simulink model "SingleTrack"  (Simulink 8.7)
settings: Solver=ode45  SolverMode=SingleTasking  StartTime=0.0  StopTime=inf  FixedStep=0.001  RelTol=1e-3
PreLoadFcn:
  | SingleTrack_params
undefined symbols (not defined in the file): Car_Bdy1_mass, Car_Steering_i, Car_Whl_Radius, Car_WhlBaseF, Car_WhlBaseR, mEngineMax, PT_DL_iDiff, PT_GearBox_iForwardGears
libraries: CarMaker4SL x7
(part 3 of 4)

== system SingleTrack/CarMaker/Vehicle/IPG Vehicle/CarAndTrailer/Forces/Tires ==
  note: The TireXX_Out signals will only be used if FileIdent is "CarMaker-Tire-CM4SL" in the tire parameter file!
      | An example parameter file can be found in Data/Tire/DT_CM4SL_UserTire.
  Sync_In : Inport
  TireFL_In : Inport  Port=2
  TireFR_In : Inport  Port=3
  TireRL_In : Inport  Port=4
  TireRR_In : Inport  Port=5
  Bus Creator{1..4} (4 alike) : BusCreator  Inputs=11
  Demux{1..3,8} (4 alike) : Demux  Outputs=7
  TireFL : Subsystem
  TireFR : Subsystem
  TireRL : Subsystem
  TireRR : Subsystem
  TireFL_Out : Outport
  TireFR_Out : Outport  Port=2
  TireRL_Out : Outport  Port=3
  TireRR_Out : Outport  Port=4
  wires:
  Sync_In/1 -> TireRR/1(Sync_In), TireRL/1(Sync_In), TireFR/1(Sync_In), TireFL/1(Sync_In)
  Bus Creator4/1 -> TireRR_Out/1
  Bus Creator2/1 -> TireRL_Out/1
  Bus Creator1/1 -> TireFR_Out/1
  Demux3/5 -> TireRR/6(Rim_turnv)  "Tire_In Rim_turnv"
  Demux3/4 -> TireRR/5(Rim_rotv)  "Tire_In Rim_rotv"
  Demux3/1 -> TireRR/2(Load)  "Tire_In Load"
  Demux3/7 -> TireRR/8(muRoad)  "Tire_In mu"
  Demux3/6 -> TireRR/7(InclinAngle)  "Tire_In Camber"
  Demux3/2 -> TireRR/3(vxtrans)  "Tire_In vxtrans"
  Demux3/3 -> TireRR/4(vytrans)  "Tire_In vytrans"
  TireRR/11(AlignTrq) -> Bus Creator4/11  "Tire_Out AlignTrq"
  TireRR/10(RollResist) -> Bus Creator4/10  "Tire_Out RollResist"
  TireRR/9(OverturnTrq) -> Bus Creator4/9  "Tire_Out OverturnTrq"
  TireRR/8(LoadFrc) -> Bus Creator4/8  "Tire_Out LoadFrc"
  TireRR/7(SideFrc) -> Bus Creator4/7  "Tire_Out SideFrc"
  TireRR/6(LongFrc) -> Bus Creator4/6  "Tire_Out LongFrc"
  TireRR/5(vBelt) -> Bus Creator4/5  "Tire_Out vBelt"
  TireRR/4(rBelt_eff) -> Bus Creator4/4  "Tire_Out rBelt_eff"
  TireRR/3(TurnSlp) -> Bus Creator4/3  "Tire_Out TurnSlp"
  TireRR/1(Slp) -> Bus Creator4/1  "Tire_Out Slp"
  TireRR/2(Alpha) -> Bus Creator4/2  "Tire_Out Alpha"
  Demux2/5 -> TireRL/6(Rim_turnv)  "Tire_In Rim_turnv"
  Demux2/4 -> TireRL/5(Rim_rotv)  "Tire_In Rim_rotv"
  Demux2/1 -> TireRL/2(Load)  "Tire_In Load"
  Demux2/7 -> TireRL/8(muRoad)  "Tire_In mu"
  Demux2/6 -> TireRL/7(InclinAngle)  "Tire_In Camber"
  Demux2/2 -> TireRL/3(vxtrans)  "Tire_In vxtrans"
  Demux2/3 -> TireRL/4(vytrans)  "Tire_In vytrans"
  TireRL/11(AlignTrq) -> Bus Creator2/11  "Tire_Out AlignTrq"
  TireRL/10(RollResist) -> Bus Creator2/10  "Tire_Out RollResist"
  TireRL/9(OverturnTrq) -> Bus Creator2/9  "Tire_Out OverturnTrq"
  TireRL/8(LoadFrc) -> Bus Creator2/8  "Tire_Out LoadFrc"
  TireRL/7(SideFrc) -> Bus Creator2/7  "Tire_Out SideFrc"
  TireRL/6(LongFrc) -> Bus Creator2/6  "Tire_Out LongFrc"
  TireRL/5(vBelt) -> Bus Creator2/5  "Tire_Out vBelt"
  TireRL/4(rBelt_eff) -> Bus Creator2/4  "Tire_Out rBelt_eff"
  TireRL/3(TurnSlp) -> Bus Creator2/3  "Tire_Out TurnSlp"
  TireRL/1(Slp) -> Bus Creator2/1  "Tire_Out Slp"
  TireRL/2(Alpha) -> Bus Creator2/2  "Tire_Out Alpha"
  Demux1/5 -> TireFR/6(Rim_turnv)  "Tire_In Rim_turnv"
  Demux1/4 -> TireFR/5(Rim_rotv)  "Tire_In Rim_rotv"
  Demux1/1 -> TireFR/2(Load)  "Tire_In Load"
  Demux1/7 -> TireFR/8(muRoad)  "Tire_In mu"
  Demux1/6 -> TireFR/7(InclinAngle)  "Tire_In Camber"
  Demux1/2 -> TireFR/3(vxtrans)  "Tire_In vxtrans"
  Demux1/3 -> TireFR/4(vytrans)  "Tire_In vytrans"
  TireFR/11(AlignTrq) -> Bus Creator1/11  "Tire_Out AlignTrq"
  TireFR/10(RollResist) -> Bus Creator1/10  "Tire_Out RollResist"
  TireFR/9(OverturnTrq) -> Bus Creator1/9  "Tire_Out OverturnTrq"
  TireFR/8(LoadFrc) -> Bus Creator1/8  "Tire_Out LoadFrc"
  TireFR/7(SideFrc) -> Bus Creator1/7  "Tire_Out SideFrc"
  TireFR/6(LongFrc) -> Bus Creator1/6  "Tire_Out LongFrc"
  TireFR/5(vBelt) -> Bus Creator1/5  "Tire_Out vBelt"
  TireFR/4(rBelt_eff) -> Bus Creator1/4  "Tire_Out rBelt_eff"
  TireFR/3(TurnSlp) -> Bus Creator1/3  "Tire_Out TurnSlp"
  TireFR/1(Slp) -> Bus Creator1/1  "Tire_Out Slp"
  TireFR/2(Alpha) -> Bus Creator1/2  "Tire_Out Alpha"
  Demux8/5 -> TireFL/6(Rim_turnv)  "Tire_In Rim_turnv"
  Demux8/4 -> TireFL/5(Rim_rotv)  "Tire_In Rim_rotv"
  TireFL_In/1 -> Demux8/1
  Demux8/1 -> TireFL/2(Load)  "Tire_In Load"
  Demux8/7 -> TireFL/8(muRoad)  "Tire_In mu"
  Demux8/6 -> TireFL/7(InclinAngle)  "Tire_In Camber"
  Demux8/2 -> TireFL/3(vxtrans)  "Tire_In vxtrans"
  Demux8/3 -> TireFL/4(vytrans)  "Tire_In vytrans"
  TireFL/11(AlignTrq) -> Bus Creator3/11  "Tire_Out AlignTrq"
  TireFL/10(RollResist) -> Bus Creator3/10  "Tire_Out RollResist"
  TireFL/9(OverturnTrq) -> Bus Creator3/9  "Tire_Out OverturnTrq"
  TireFL/8(LoadFrc) -> Bus Creator3/8  "Tire_Out LoadFrc"
  TireFL/7(SideFrc) -> Bus Creator3/7  "Tire_Out SideFrc"
  TireFL/6(LongFrc) -> Bus Creator3/6  "Tire_Out LongFrc"
  TireFL/5(vBelt) -> Bus Creator3/5  "Tire_Out vBelt"
  TireFL/4(rBelt_eff) -> Bus Creator3/4  "Tire_Out rBelt_eff"
  TireFL/3(TurnSlp) -> Bus Creator3/3  "Tire_Out TurnSlp"
  TireFL/1(Slp) -> Bus Creator3/1  "Tire_Out Slp"
  TireFL/2(Alpha) -> Bus Creator3/2  "Tire_Out Alpha"
  Bus Creator3/1 -> TireFL_Out/1
  TireFR_In/1 -> Demux1/1
  TireRL_In/1 -> Demux2/1
  TireRR_In/1 -> Demux3/1

== system SingleTrack/CarMaker/Vehicle/IPG Vehicle/CarAndTrailer/Forces/Vehicle Forces ==
  Sync_In : Inport
  Bus Creator1 : BusCreator  Inputs=12
  Bus Creator8 : BusCreator  Inputs=16
  BusCreator1 : BusCreator  Inputs=4
  BusCreator2 : BusCreator  Inputs=9
  Demux : Demux  Outputs=16
  Demux1 : Demux  Outputs=12
  Demux2 : Demux  Outputs=13
  Forces : S-Function  FunctionName=CM_Sfun  Parameters='Forces'  SFunctionDeploymentMode=off  EnableBusSupport=off
  Terminator : Terminator
  Sync_Out : Outport
  Car.Virtual : Outport  Port=2
  Car.Aero : Outport  Port=3
  Car.Load : Outport  Port=4
  wires:
  BusCreator1/1 -> Terminator/1  "Aero IF (in)"
  Demux2/13 -> BusCreator2/9  "car Aero Trq_1 z"
  Demux2/12 -> BusCreator2/8  "car Aero Trq_1 y"
  Demux2/11 -> BusCreator2/7  "car Aero Trq_1 x"
  Demux2/10 -> BusCreator2/6  "car Aero Frc_1 z"
  Demux2/9 -> BusCreator2/5  "car Aero Frc_1 y"
  Demux2/8 -> BusCreator2/4  "car Aero Frc_1 x"
  Demux2/7 -> BusCreator2/3  "car Aero PoA_1 z"
  Demux2/6 -> BusCreator2/2  "car Aero PoA_1 y"
  Demux2/5 -> BusCreator2/1  "car Aero PoA_1 x"
  Demux2/4 -> BusCreator1/4  "car Aero tau_1"
  Demux2/3 -> BusCreator1/3  "car Aero ApproachVel_1 z"
  Demux2/2 -> BusCreator1/2  "car Aero ApproachVel_1 y"
  Demux2/1 -> BusCreator1/1  "car Aero ApproachVel_1 x"
  Demux/16 -> Bus Creator8/16  "Car Load_3 tz"
  Demux/15 -> Bus Creator8/15  "Car Load_3 ty"
  Demux/14 -> Bus Creator8/14  "Car Load_3 tx"
  Demux/13 -> Bus Creator8/13  "Car Load_3 mass"
  Demux1/12 -> Bus Creator1/12  "Car Virtual Trq_0 z"
  Demux1/11 -> Bus Creator1/11  "Car Virtual Trq_0 y"
  Demux1/10 -> Bus Creator1/10  "Car Virtual Trq_0 x"
  Demux1/9 -> Bus Creator1/9  "Car Virtual Trq_1 z"
  Demux1/8 -> Bus Creator1/8  "Car Virtual Trq_1 y"
  Demux1/7 -> Bus Creator1/7  "Car Virtual Trq_1 x"
  Demux1/6 -> Bus Creator1/6  "Car Virtual Frc_0 z"
  Demux1/5 -> Bus Creator1/5  "Car Virtual Frc_0 y"
  Demux1/4 -> Bus Creator1/4  "Car Virtual Frc_0 x"
  Sync_In/1 -> Forces/1
  Forces/1 -> Sync_Out/1
  BusCreator2/1 -> Car.Aero/1
  Demux1/1 -> Bus Creator1/1  "Car Virtual Frc_1 x"
  Demux1/2 -> Bus Creator1/2  "Car Virtual Frc_1 y"
  Demux1/3 -> Bus Creator1/3  "Car Virtual Frc_1 z"
  Forces/3 -> Demux2/1
  Forces/2 -> Demux1/1
  Bus Creator1/1 -> Car.Virtual/1
  Bus Creator8/1 -> Car.Load/1
  Demux/1 -> Bus Creator8/1  "Car Load_0 mass"
  Demux/2 -> Bus Creator8/2  "Car Load_0 tx"
  Demux/3 -> Bus Creator8/3  "Car Load_0 ty"
  Demux/4 -> Bus Creator8/4  "Car Load_0 tz"
  Demux/5 -> Bus Creator8/5  "Car Load_1 mass"
  Demux/6 -> Bus Creator8/6  "Car Load_1 tx"
  Demux/7 -> Bus Creator8/7  "Car Load_1 ty"
  Demux/8 -> Bus Creator8/8  "Car Load_1 tz"
  Demux/9 -> Bus Creator8/9  "Car Load_2 mass"
  Demux/10 -> Bus Creator8/10  "Car Load_2 tx"
  Demux/11 -> Bus Creator8/11  "Car Load_2 ty"
  Demux/12 -> Bus Creator8/12  "Car Load_2 tz"
  Forces/4 -> Demux/1

== system SingleTrack/CarMaker/Vehicle/IPG Vehicle/CarAndTrailer/Trailer/CreateBus Car.Hitch.FrcTrq ==
  In1 : Inport
  Bus Creator7 : BusCreator  Inputs=6
  Demux7 : Demux  Outputs=6
  Out1 : Outport
  wires:
  In1/1 -> Demux7/1
  Bus Creator7/1 -> Out1/1
  Demux7/6 -> Bus Creator7/6  "Car Hitch Trq2Car z"
  Demux7/5 -> Bus Creator7/5  "Car Hitch Trq2Car y"
  Demux7/4 -> Bus Creator7/4  "Car Hitch Trq2Car x"
  Demux7/3 -> Bus Creator7/3  "Car Hitch Frc2Car z"
  Demux7/2 -> Bus Creator7/2  "Car Hitch Frc2Car y"
  Demux7/1 -> Bus Creator7/1  "Car Hitch Frc2Car x"

== system SingleTrack/CarMaker/Vehicle/IPG Vehicle/CarAndTrailer/Trailer/CreateBus Vhcl.Motion ==
  In1 : Inport
  BusCreator : BusCreator  Inputs=15
  Demux : Demux  Outputs=15
  Out1 : Outport
  wires:
  Demux/15 -> BusCreator/15  "Vhcl YawAcc"
  Demux/14 -> BusCreator/14  "Vhcl YawVel"
  Demux/13 -> BusCreator/13  "Vhcl Yaw"
  Demux/12 -> BusCreator/12  "Vhcl PitchAcc"
  Demux/11 -> BusCreator/11  "Vhcl PitchVel"
  Demux/10 -> BusCreator/10  "Vhcl Pitch"
  Demux/9 -> BusCreator/9  "Vhcl RollAcc"
  Demux/8 -> BusCreator/8  "Vhcl RollVel"
  Demux/7 -> BusCreator/7  "Vhcl Roll"
  Demux/6 -> BusCreator/6  "Vhcl Hitch_Pos z"
  Demux/5 -> BusCreator/5  "Vhcl Hitch_Pos y"
  Demux/4 -> BusCreator/4  "Vhcl Hitch_Pos x"
  Demux/3 -> BusCreator/3  "Vhcl sRoad"
  Demux/2 -> BusCreator/2  "Vhcl Distance"
  Demux/1 -> BusCreator/1  "Vhcl v"
  In1/1 -> Demux/1
  BusCreator/1 -> Out1/1

== system SingleTrack/CarMaker/Vehicle/IPG Vehicle/CarAndTrailer/Trailer/CreateBus Vhcl.PoI ==
  In1 : Inport
  Bus Creator3 : BusCreator  Inputs=18
  Demux3 : Demux  Outputs=18
  Out1 : Outport
  wires:
  Demux3/18 -> Bus Creator3/18  "Vhcl PoI_GCS Elev"
  Demux3/17 -> Bus Creator3/17  "Vhcl PoI_GCS Lat"
  Demux3/16 -> Bus Creator3/16  "Vhcl PoI_GCS Long"
  Demux3/15 -> Bus Creator3/15  "Vhcl PoI_Acc_1 z"
  Demux3/14 -> Bus Creator3/14  "Vhcl PoI_Acc_1 y"
  Demux3/13 -> Bus Creator3/13  "Vhcl PoI_Acc_1 x"
  Demux3/12 -> Bus Creator3/12  "Vhcl PoI_Vel_1 z"
  Demux3/11 -> Bus Creator3/11  "Vhcl PoI_Vel_1 y"
  Demux3/10 -> Bus Creator3/10  "Vhcl PoI_Vel_1 x"
  Demux3/9 -> Bus Creator3/9  "Vhcl PoI_Acc z"
  Demux3/8 -> Bus Creator3/8  "Vhcl PoI_Acc y"
  Demux3/7 -> Bus Creator3/7  "Vhcl PoI_Acc x"
  Demux3/6 -> Bus Creator3/6  "Vhcl PoI_Vel z"
  Demux3/5 -> Bus Creator3/5  "Vhcl PoI_Vel y"
  Demux3/4 -> Bus Creator3/4  "Vhcl PoI_Vel x"
  Demux3/3 -> Bus Creator3/3  "Vhcl PoI_Pos z"
  Demux3/2 -> Bus Creator3/2  "Vhcl PoI_Pos y"
  In1/1 -> Demux3/1
  Bus Creator3/1 -> Out1/1
  Demux3/1 -> Bus Creator3/1  "Vhcl PoI_Pos x"

== system SingleTrack/CarMaker/Vehicle/IPG Vehicle/CarAndTrailer/Trailer/CreateBus Vhcl.Steering ==
  In1 : Inport
  Bus Creator3 : BusCreator  Inputs=4
  Demux : Demux
  Out1 : Outport
  wires:
  Bus Creator3/1 -> Out1/1
  Demux/1 -> Bus Creator3/1  "Vhcl Steering Ang"
  Demux/3 -> Bus Creator3/3  "Vhcl Steering AngAcc"
  Demux/2 -> Bus Creator3/2  "Vhcl Steering AngVel"
  Demux/4 -> Bus Creator3/4  "Vhcl Steering Trq"
  In1/1 -> Demux/1

== system SingleTrack/CarMaker/Vehicle/IPG Vehicle/CarAndTrailer/Trailer/CreateBus Vhcl.Wheel.FL ==
  In1 : Inport
  Bus Creator3 : BusCreator  Inputs=14
  Demux3 : Demux  Outputs=14
  Out1 : Outport
  wires:
  Demux3/14 -> Bus Creator3/14  "Vhcl Wheel FL Trq_WhlBearing"
  Demux3/13 -> Bus Creator3/13  "Vhcl Wheel FL Trq_T2W"
  Demux3/12 -> Bus Creator3/12  "Vhcl Wheel FL SideSlip"
  Demux3/11 -> Bus Creator3/11  "Vhcl Wheel FL LongSlip"
  Demux3/10 -> Bus Creator3/10  "Vhcl Wheel FL vBelt"
  Demux3/9 -> Bus Creator3/9  "Vhcl Wheel FL Fz"
  Demux3/8 -> Bus Creator3/8  "Vhcl Wheel FL Fy"
  Demux3/7 -> Bus Creator3/7  "Vhcl Wheel FL Fx"
  Demux3/6 -> Bus Creator3/6  "Vhcl Wheel FL r_zxy z"
  Demux3/5 -> Bus Creator3/5  "Vhcl Wheel FL r_zxy y"
  Demux3/4 -> Bus Creator3/4  "Vhcl Wheel FL r_zxy x"
  Demux3/3 -> Bus Creator3/3  "Vhcl Wheel FL t z"
  Demux3/2 -> Bus Creator3/2  "Vhcl Wheel FL t y"
  In1/1 -> Demux3/1
  Bus Creator3/1 -> Out1/1
  Demux3/1 -> Bus Creator3/1  "Vhcl Wheel FL t x"

== system SingleTrack/CarMaker/Vehicle/IPG Vehicle/CarAndTrailer/Trailer/CreateBus Vhcl.Wheel.FR ==
  In1 : Inport
  Bus Creator3 : BusCreator  Inputs=14
  Demux3 : Demux  Outputs=14
  Out1 : Outport
  wires:
  Demux3/14 -> Bus Creator3/14  "Vhcl Wheel FR Trq_WhlBearing"
  Demux3/13 -> Bus Creator3/13  "Vhcl Wheel FR Trq_T2W"
  Demux3/12 -> Bus Creator3/12  "Vhcl Wheel FR SideSlip"
  Demux3/11 -> Bus Creator3/11  "Vhcl Wheel FR LongSlip"
  Demux3/10 -> Bus Creator3/10  "Vhcl Wheel FR vBelt"
  Demux3/9 -> Bus Creator3/9  "Vhcl Wheel FR Fz"
  Demux3/8 -> Bus Creator3/8  "Vhcl Wheel FR Fy"
  Demux3/7 -> Bus Creator3/7  "Vhcl Wheel FR Fx"
  Demux3/6 -> Bus Creator3/6  "Vhcl Wheel FR r_zxy z"
  Demux3/5 -> Bus Creator3/5  "Vhcl Wheel FR r_zxy y"
  Demux3/4 -> Bus Creator3/4  "Vhcl Wheel FR r_zxy x"
  Demux3/3 -> Bus Creator3/3  "Vhcl Wheel FR t z"
  Demux3/2 -> Bus Creator3/2  "Vhcl Wheel FR t y"
  In1/1 -> Demux3/1
  Bus Creator3/1 -> Out1/1
  Demux3/1 -> Bus Creator3/1  "Vhcl Wheel FR t x"

== system SingleTrack/CarMaker/Vehicle/IPG Vehicle/CarAndTrailer/Trailer/CreateBus Vhcl.Wheel.RL ==
  In1 : Inport
  Bus Creator3 : BusCreator  Inputs=14
  Demux3 : Demux  Outputs=14
  Out1 : Outport
  wires:
  Demux3/14 -> Bus Creator3/14  "Vhcl Wheel RL Trq_WhlBearing"
  Demux3/13 -> Bus Creator3/13  "Vhcl Wheel RL Trq_T2W"
  Demux3/12 -> Bus Creator3/12  "Vhcl Wheel RL SideSlip"
  Demux3/11 -> Bus Creator3/11  "Vhcl Wheel RL LongSlip"
  Demux3/10 -> Bus Creator3/10  "Vhcl Wheel RL vBelt"
  Demux3/9 -> Bus Creator3/9  "Vhcl Wheel RL Fz"
  Demux3/8 -> Bus Creator3/8  "Vhcl Wheel RL Fy"
  Demux3/7 -> Bus Creator3/7  "Vhcl Wheel RL Fx"
  Demux3/6 -> Bus Creator3/6  "Vhcl Wheel RL r_zxy z"
  Demux3/5 -> Bus Creator3/5  "Vhcl Wheel RL r_zxy y"
  Demux3/4 -> Bus Creator3/4  "Vhcl Wheel RL r_zxy x"
  Demux3/3 -> Bus Creator3/3  "Vhcl Wheel RL t z"
  Demux3/2 -> Bus Creator3/2  "Vhcl Wheel RL t y"
  In1/1 -> Demux3/1
  Bus Creator3/1 -> Out1/1
  Demux3/1 -> Bus Creator3/1  "Vhcl Wheel RL t x"

== system SingleTrack/CarMaker/Vehicle/IPG Vehicle/CarAndTrailer/Trailer/CreateBus Vhcl.Wheel.RR ==
  In1 : Inport
  Bus Creator3 : BusCreator  Inputs=14
  Demux3 : Demux  Outputs=14
  Out1 : Outport
  wires:
  Demux3/14 -> Bus Creator3/14  "Vhcl Wheel RR Trq_WhlBearing"
  Demux3/13 -> Bus Creator3/13  "Vhcl Wheel RR Trq_T2W"
  Demux3/12 -> Bus Creator3/12  "Vhcl Wheel RR SideSlip"
  Demux3/11 -> Bus Creator3/11  "Vhcl Wheel RR LongSlip"
  Demux3/10 -> Bus Creator3/10  "Vhcl Wheel RR vBelt"
  Demux3/9 -> Bus Creator3/9  "Vhcl Wheel RR Fz"
  Demux3/8 -> Bus Creator3/8  "Vhcl Wheel RR Fy"
  Demux3/7 -> Bus Creator3/7  "Vhcl Wheel RR Fx"
  Demux3/6 -> Bus Creator3/6  "Vhcl Wheel RR r_zxy z"
  Demux3/5 -> Bus Creator3/5  "Vhcl Wheel RR r_zxy y"
  Demux3/4 -> Bus Creator3/4  "Vhcl Wheel RR r_zxy x"
  Demux3/3 -> Bus Creator3/3  "Vhcl Wheel RR t z"
  Demux3/2 -> Bus Creator3/2  "Vhcl Wheel RR t y"
  In1/1 -> Demux3/1
  Bus Creator3/1 -> Out1/1
  Demux3/1 -> Bus Creator3/1  "Vhcl Wheel RR t x"

== system SingleTrack/CarMaker/Vehicle/User Vehicle (CM4SL)/CarAndTrailer/CarAndTrailerUpd/CreateBus Brake.IF.In ==
  In : Inport
  BusCreator : BusCreator  Inputs=9
  Demux : Demux  Outputs=9
  Out : Outport
  wires:
  Demux/9 -> BusCreator/9  "Brake IF Trq_Reg RR"
  Demux/8 -> BusCreator/8  "Brake IF Trq_Reg RL"
  Demux/7 -> BusCreator/7  "Brake IF Trq_Reg FR"
  Demux/6 -> BusCreator/6  "Brake IF Trq_Reg FL"
  Demux/5 -> BusCreator/5  "Brake IF Trq_Reg_max RR"
  Demux/4 -> BusCreator/4  "Brake IF Trq_Reg_max RL"
  Demux/3 -> BusCreator/3  "Brake IF Trq_Reg_max FR"
  Demux/2 -> BusCreator/2  "Brake IF Trq_Reg_max FL"
  Demux/1 -> BusCreator/1  "Brake IF T_env"
  BusCreator/1 -> Out/1
  In/1 -> Demux/1

== system SingleTrack/CarMaker/Vehicle/User Vehicle (CM4SL)/CarAndTrailer/CreateBus Vhcl.Fr1/BdyFrame2Vhcl.Fr1A ==
  note: Translate pseudo BdyFrame interface to Vhcl.Fr1
  t_0 : Inport
  v_0 : Inport  Port=2
  a_0 : Inport  Port=3
  omega_0 : Inport  Port=4
  alpha_0 : Inport  Port=5
  Tr2Fr0 : Inport  Port=6
  Bus Creator : BusCreator  Inputs=24
  Demux{,1..3,5} (5 alike) : Demux  Outputs=3
  Demux4 : Demux  Outputs=9
  Vhcl.Fr1 : Outport
  wires:
  t_0/1 -> Demux/1
  v_0/1 -> Demux1/1
  a_0/1 -> Demux2/1
  omega_0/1 -> Demux3/1
  alpha_0/1 -> Demux5/1
  Tr2Fr0/1 -> Demux4/1
  Demux4/9 -> Bus Creator/24  "Vhcl Fr1A_Tr2Fr0 22"
  Demux4/8 -> Bus Creator/23  "Vhcl Fr1A_Tr2Fr0 21"
  Demux4/7 -> Bus Creator/22  "Vhcl Fr1A_Tr2Fr0 20"
  Demux4/6 -> Bus Creator/21  "Vhcl Fr1A_Tr2Fr0 12"
  Demux4/5 -> Bus Creator/20  "Vhcl Fr1A_Tr2Fr0 11"
  Demux4/4 -> Bus Creator/19  "Vhcl Fr1A_Tr2Fr0 10"
  Demux4/3 -> Bus Creator/18  "Vhcl Fr1A_Tr2Fr0 02"
  Demux4/2 -> Bus Creator/17  "Vhcl Fr1A_Tr2Fr0 01"
  Demux4/1 -> Bus Creator/16  "Vhcl Fr1A_Tr2Fr0 00"
  Demux5/3 -> Bus Creator/15  "Vhcl Fr1A_alpha_0 z"
  Demux5/2 -> Bus Creator/14  "Vhcl Fr1A_alpha_0 y"
  Demux5/1 -> Bus Creator/13  "Vhcl Fr1A_alpha_0 x"
  Demux3/3 -> Bus Creator/12  "Vhcl Fr1A_omega_0 z"
  Demux3/2 -> Bus Creator/11  "Vhcl Fr1A_omega_0 y"
  Demux3/1 -> Bus Creator/10  "Vhcl Fr1A_omega_0 x"
  Demux2/3 -> Bus Creator/9  "Vhcl Fr1A_a_0 z"
  Demux2/2 -> Bus Creator/8  "Vhcl Fr1A_a_0 y"
  Demux2/1 -> Bus Creator/7  "Vhcl Fr1A_a_0 x"
  Demux1/3 -> Bus Creator/6  "Vhcl Fr1A_v_0 z"
  Demux1/2 -> Bus Creator/5  "Vhcl Fr1A_v_0 y"
  Demux1/1 -> Bus Creator/4  "Vhcl Fr1A_v_0 x"
  Demux/3 -> Bus Creator/3  "Vhcl Fr1A_t_0 z"
  Demux/2 -> Bus Creator/2  "Vhcl Fr1A_t_0 y"
  Demux/1 -> Bus Creator/1  "Vhcl Fr1 A_t_0 x"
  Bus Creator/1 -> Vhcl.Fr1/1

== system SingleTrack/CarMaker/Vehicle/User Vehicle (CM4SL)/CarAndTrailer/CreateBus Vhcl.Fr1/Tr2Fr0 ==
  Car : Inport
  Bus Creator : BusCreator  Inputs=9
  Subsystem_00 : Subsystem
  Subsystem_01 : Subsystem
  Subsystem_02 : Subsystem
  Subsystem_10 : Subsystem
  Subsystem_11 : Subsystem
  Subsystem_12 : Subsystem
  Subsystem_20 : Subsystem
  Subsystem_21 : Subsystem
  Subsystem_22 : Subsystem
  sincos : Subsystem
  Tr2Fr0 : Outport
  wires:
  Car/1 -> sincos/1(Car)
  sincos/1(sincos) -> Subsystem_10/1(sincos), Subsystem_11/1(sincos), Subsystem_20/1(sincos), Subsystem_21/1(sincos), Subsystem_22/1(sincos), Subsystem_12/1(sincos), Subsystem_00/1(sincos), Subsystem_01/1(sincos), Subsystem_02/1(sincos)
  Bus Creator/1 -> Tr2Fr0/1
  Subsystem_00/1(Tr2Fr1_00) -> Bus Creator/1  "Tr2Fr0_00"
  Subsystem_10/1(Tr2Fr1_10) -> Bus Creator/4  "Tr2Fr0_10"
  Subsystem_20/1(Tr2Fr1_20) -> Bus Creator/7  "Tr2Fr0_20"
  Subsystem_21/1(Tr2Fr1_21) -> Bus Creator/8  "Tr2Fr0_21"
  Subsystem_22/1(Tr2Fr1_22) -> Bus Creator/9  "Tr2Fr0_22"
  Subsystem_01/1(Tr2Fr1_01) -> Bus Creator/2  "Tr2Fr0_01"
  Subsystem_02/1(Tr2Fr1_02) -> Bus Creator/3  "Tr2Fr0_02"
  Subsystem_11/1(Tr2Fr1_11) -> Bus Creator/5  "Tr2Fr1_11"
  Subsystem_12/1(Tr2Fr1_12) -> Bus Creator/6  "Tr2Fr1_12"

== system SingleTrack/CarMaker/Vehicle/User Vehicle (CM4SL)/CarAndTrailer/CreateBus Vhcl.Fr1/a_0 ==
  Car : Inport
  Tr2Fr0 : Inport  Port=2
  Add : Sum
  Add1 : Sum
  Add2 : Sum
  Bus Selector1 : BusSelector  OutputSignals=Car_ax_1,Car_ay_1
  Bus Selector2 : BusSelector  OutputSignals=Tr2Fr0_00,Tr2Fr0_01,Tr2Fr0_10,Tr2Fr1_11,Tr2Fr0_20,Tr2Fr0_21
  Mux1 : Mux  Inputs=3
  Product{,1..5} (6 alike) : Product  RndMeth=Zero
  a_0 : Outport
  wires:
  Mux1/1 -> a_0/1
  Car/1 -> Bus Selector1/1
  Tr2Fr0/1 -> Bus Selector2/1
  Bus Selector1/2 -> Product/1, Product2/1, Product4/1  "<Car_ay_1>"
  Bus Selector1/1 -> Product1/1, Product3/1, Product5/1  "<Car_ax_1>"
  Product1/1 -> Add/1
  Product/1 -> Add/2
  Add/1 -> Mux1/1
  Product3/1 -> Add1/1
  Product2/1 -> Add1/2
  Bus Selector2/1 -> Product1/2  "<Tr2Fr0_00>"
  Bus Selector2/2 -> Product/2  "<Tr2Fr0_01>"
  Add1/1 -> Mux1/2
  Bus Selector2/3 -> Product3/2  "<Tr2Fr0_10>"
  Bus Selector2/4 -> Product2/2  "<Tr2Fr1_11>"
  Product5/1 -> Add2/1
  Product4/1 -> Add2/2
  Add2/1 -> Mux1/3
  Bus Selector2/6 -> Product4/2  "<Tr2Fr0_21>"
  Bus Selector2/5 -> Product5/2  "<Tr2Fr0_20>"

== system SingleTrack/CarMaker/Vehicle/User Vehicle (CM4SL)/CarAndTrailer/CreateBus Vhcl.Fr1/t_0 ==
  Car : Inport
  Bus Selector : BusSelector  OutputSignals=Car_x,Car_y,Road_Fr1_z
  Mux : Mux  Inputs=3
  t_0 : Outport
  wires:
  Bus Selector/1 -> Mux/1  "<Car_x>"
  Bus Selector/2 -> Mux/2  "<Car_y>"
  Bus Selector/3 -> Mux/3  "<Road_Fr1_z>"
  Car/1 -> Bus Selector/1
  Mux/1 -> t_0/1

== system SingleTrack/CarMaker/Vehicle/User Vehicle (CM4SL)/CarAndTrailer/CreateBus Vhcl.Fr1/v_0 ==
  Car : Inport
  Tr2Fr0 : Inport  Port=2
  Bus Selector1 : BusSelector  OutputSignals=Car_vx_1
  Bus Selector2 : BusSelector  OutputSignals=Tr2Fr0_00,Tr2Fr0_10,Tr2Fr0_20
  Mux1 : Mux  Inputs=3
  Product : Product  RndMeth=Zero
  Product1 : Product  RndMeth=Zero
  Product2 : Product  RndMeth=Zero
  v_0 : Outport
  wires:
  Car/1 -> Bus Selector1/1
  Mux1/1 -> v_0/1
  Tr2Fr0/1 -> Bus Selector2/1
  Bus Selector2/1 -> Product/2  "<Tr2Fr0_00>"
  Bus Selector2/2 -> Product1/2  "<Tr2Fr0_10>"
  Bus Selector2/3 -> Product2/2  "<Tr2Fr0_20>"
  Bus Selector1/1 -> Product/1, Product1/1, Product2/1  "<Car_vx_1>"
  Product/1 -> Mux1/1
  Product1/1 -> Mux1/2
  Product2/1 -> Mux1/3

== system SingleTrack/CarMaker/Vehicle/User Vehicle (CM4SL)/CarAndTrailer/PowerTrainUpd/Set OperationState ==
  note: Handles OperationState in Post-processing (SimCore.State >=9)
  If : If  IfExpression=u1 >= 9
  If Action Subsystem : Subsystem  TreatAsAtomicUnit=on
  If Action Subsystem1 : Subsystem  TreatAsAtomicUnit=on
  Merge : Merge
  Read CM Dict : CarMaker4SL/Read CM Dict  xname=SC.State  xsync=off
  Read CM Dict1 : CarMaker4SL/Read CM Dict  xname=DM.OperationState_trg  xsync=off
  OperationState : Outport
  wires:
  Merge/1 -> OperationState/1
  If/1 -> If Action Subsystem/Action
  If/2 -> If Action Subsystem1/Action
  If Action Subsystem/1(Out1) -> Merge/1
  If Action Subsystem1/1(Out1) -> Merge/2
  Read CM Dict/1 -> If/1
  Read CM Dict1/1 -> If Action Subsystem1/1(In1), If Action Subsystem/1(In1)

== system SingleTrack/CarMaker/Vehicle/User Vehicle (CM4SL)/CarAndTrailer/Query Road/IPGRoad5 ==
  rIn.st : Inport
  rIn.xyz : Inport  Port=2
  Bus Creator1 : BusCreator  Inputs=9
  Bus Creator2 : BusCreator  Inputs=22
  Demux1 : Demux  Outputs=9
  Demux3 : Demux  Outputs=22
  S-Function : S-Function  FunctionName=cm_road  Parameters=xname,xevalmode,xconsiderbumps,xusepath,xwithcurve,xabort  SFunctionDeploymentMode=off  EnableBusSupport=off
  rOutGeo : Outport
  rOutRoute : Outport  Port=2
  wires:
  Demux3/22 -> Bus Creator2/22  "fric"
  S-Function/2 -> Demux3/1
  S-Function/1 -> Demux1/1
  Bus Creator1/1 -> rOutGeo/1
  Demux1/9 -> Bus Creator1/9  "fric"
  Demux1/8 -> Bus Creator1/8  "onJunction"
  Demux1/7 -> Bus Creator1/7  "onRoad"
  Demux1/6 -> Bus Creator1/6  "nuv z"
  Demux1/5 -> Bus Creator1/5  "nuv y"
  Demux1/4 -> Bus Creator1/4  "nuv x"
  Demux1/3 -> Bus Creator1/3  "z"
  Demux1/2 -> Bus Creator1/2  "y"
  Demux1/1 -> Bus Creator1/1  "x"
  Demux3/21 -> Bus Creator2/21  "curveZ"
  Demux3/20 -> Bus Creator2/20  "slope"
  Demux3/19 -> Bus Creator2/19  "grade"
  Demux3/18 -> Bus Creator2/18  "onRoad"
  Demux3/17 -> Bus Creator2/17  "width right"
  Demux3/16 -> Bus Creator2/16  "width left"
  Demux3/15 -> Bus Creator2/15  "curveXY"
  Demux3/13 -> Bus Creator2/13  "s"
  Demux3/14 -> Bus Creator2/14  "t"
  Demux3/12 -> Bus Creator2/12  "tuv z"
  Demux3/11 -> Bus Creator2/11  "tuv y"
  Demux3/10 -> Bus Creator2/10  "tuv x"
  Demux3/9 -> Bus Creator2/9  "suv z"
  Demux3/8 -> Bus Creator2/8  "suv y"
  Demux3/7 -> Bus Creator2/7  "suv x"
  Demux3/6 -> Bus Creator2/6  "nuv z"
  Demux3/5 -> Bus Creator2/5  "nuv y"
  Demux3/4 -> Bus Creator2/4  "nuv x"
  Demux3/3 -> Bus Creator2/3  "z"
  Demux3/2 -> Bus Creator2/2  "y"
  Demux3/1 -> Bus Creator2/1  "x"
  Bus Creator2/1 -> rOutRoute/1
  rIn.xyz/1 -> S-Function/2
  rIn.st/1 -> S-Function/1

== system SingleTrack/CarMaker/Vehicle/User Vehicle (CM4SL)/CarAndTrailer/single-track mass point model/Car.v_1 ==
  ax : Inport
  Constant1 : Constant  Value=0.1
  PassIfSim : Subsystem
  Read CM Parameter : CarMaker4SL/Read CM Parameter  xfile=Testrun  xkey=DrivMan.Init.Velocity  xnout=1  xdefaults=0  xmuxed=on
  kmh2ms : Gain  Gain=1000/3600  OutDataTypeStr=Inherit: Inherit via back propagation  SaturateOnIntegerOverflow=on  ParamDataTypeStr=Inherit: Same as input
  vMin : MinMax  Function=max  Inputs=2  SaturateOnIntegerOverflow=on  InputSameDT=on
  v_dot * dt : Integrator  ExternalReset=level  InitialConditionSource=external  InitialCondition=22.222
  v_1 : Outport
  wires:
  Read CM Parameter/1 -> kmh2ms/1
  kmh2ms/1 -> vMin/2
  Constant1/1 -> vMin/1
  [TRStart] -> v_dot * dt/2
  vMin/1 -> v_dot * dt/3
  v_dot * dt/1 -> v_1/1
  ax/1 -> PassIfSim/1(In1)
  PassIfSim/1(Out1) -> v_dot * dt/1

== system SingleTrack/CarMaker/Vehicle/User Vehicle (CM4SL)/CarAndTrailer/single-track mass point model/PassIfSim ==
  note: Output original value only when simulating,
      | and zero during pre- or postprocessing.
  In1 : Inport
  "   " : Product  SaturateOnIntegerOverflow=on  InputSameDT=on  OutDataTypeStr=Inherit: Same as first input
  Data Type Conversion : DataTypeConversion
  Out1 : Outport
  wires:
  [TRSim] -> Data Type Conversion/1
  "   "/1 -> Out1/1
  Data Type Conversion/1 -> "   "/2
  In1/1 -> "   "/1

== system SingleTrack/CarMaker/Vehicle/User Vehicle (CM4SL)/CarAndTrailer/single-track mass point model/PassIfSim1 ==
  note: Output original value only when simulating,
      | and zero during pre- or postprocessing.
  In1 : Inport
  "   " : Product  SaturateOnIntegerOverflow=on  InputSameDT=on  OutDataTypeStr=Inherit: Same as first input
  Data Type Conversion : DataTypeConversion
  Out1 : Outport
  wires:
  [TRSim] -> Data Type Conversion/1
  "   "/1 -> Out1/1
  Data Type Conversion/1 -> "   "/2
  In1/1 -> "   "/1

== system SingleTrack/CarMaker/Vehicle/User Vehicle (CM4SL)/CarAndTrailer/single-track mass point model/PassIfSim2 ==
  note: Output original value only when simulating,
      | and zero during pre- or postprocessing.
  In1 : Inport
  "   " : Product  SaturateOnIntegerOverflow=on  InputSameDT=on  OutDataTypeStr=Inherit: Same as first input
  Data Type Conversion : DataTypeConversion
  Out1 : Outport
  wires:
  [TRSim] -> Data Type Conversion/1
  "   "/1 -> Out1/1
  Data Type Conversion/1 -> "   "/2
  In1/1 -> "   "/1

== system SingleTrack/CarMaker/Vehicle/User Vehicle (CM4SL)/CarAndTrailer/single-track mass point model/Vehicle Initial Cfg ==
  CreateBus Vhcl.Cfg : Subsystem
  VehicleControlUpd : S-Function  FunctionName=cm_initial  SFunctionDeploymentMode=off  EnableBusSupport=off
  Vhcl.Cfg : Outport
  wires:
  VehicleControlUpd/1 -> CreateBus Vhcl.Cfg/1(In1)
  CreateBus Vhcl.Cfg/1(Out1) -> Vhcl.Cfg/1

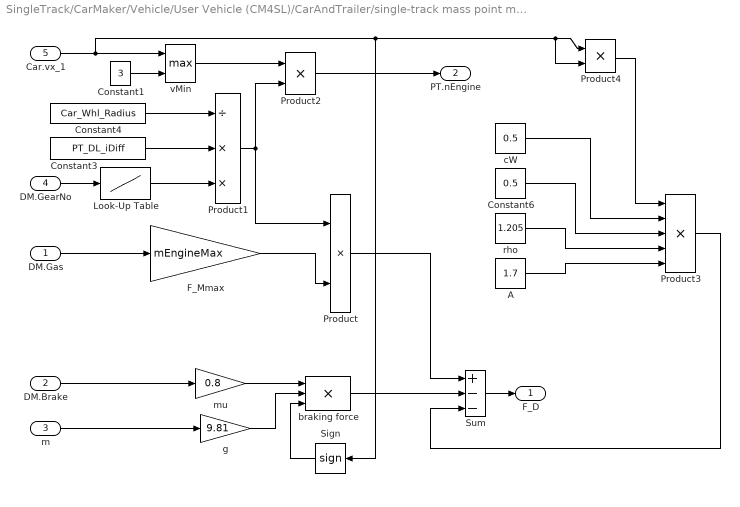
== system SingleTrack/CarMaker/Vehicle/User Vehicle (CM4SL)/CarAndTrailer/single-track mass point model/driving force ==
  DM.Gas : Inport
  DM.Brake : Inport  Port=2
  m : Inport  Port=3
  DM.GearNo : Inport  Port=4
  Car.vx_1 : Inport  Port=5
  A : Constant  Value=1.7
  Constant1 : Constant  Value=3
  Constant3 : Constant  Value=PT_DL_iDiff
  Constant4 : Constant  Value=Car_Whl_Radius
  Constant6 : Constant  Value=0.5
  "F_Mmax " : Gain  Gain=mEngineMax  SaturateOnIntegerOverflow=on  OutDataTypeStr=Inherit: Same as input  ParamDataTypeStr=Inherit: Same as input
  Look-Up Table : Lookup  InputValues=[0 1 2 3 4 5 6]  Table=PT_GearBox_iForwardGears  LookUpMeth=Interpolation-Use End Values  SaturateOnIntegerOverflow=on
  Product : Product  Inputs=**  SaturateOnIntegerOverflow=on  InputSameDT=on  OutDataTypeStr=Inherit: Same as first input
  Product1 : Product  Inputs=/**  SaturateOnIntegerOverflow=on  InputSameDT=on  OutDataTypeStr=Inherit: Same as first input
  Product2 : Product  SaturateOnIntegerOverflow=on  InputSameDT=on  OutDataTypeStr=Inherit: Same as first input
  Product3 : Product  Inputs=5  SaturateOnIntegerOverflow=on  InputSameDT=on  OutDataTypeStr=Inherit: Same as first input
  Product4 : Product  SaturateOnIntegerOverflow=on  InputSameDT=on  OutDataTypeStr=Inherit: Same as first input
  Sign : Signum  ZeroCross=off
  Sum : Sum  Inputs=+--  SaturateOnIntegerOverflow=on  InputSameDT=on  OutDataTypeStr=Inherit: Same as first input
  braking force : Product  Inputs=3  SaturateOnIntegerOverflow=on  InputSameDT=on  OutDataTypeStr=Inherit: Same as first input
  cW : Constant  Value=0.5
  g : Gain  Gain=9.81  SaturateOnIntegerOverflow=on  OutDataTypeStr=Inherit: Same as input  ParamDataTypeStr=Inherit: Same as input
  mu : Gain  Gain=0.8  SaturateOnIntegerOverflow=on  OutDataTypeStr=Inherit: Same as input  ParamDataTypeStr=Inherit: Same as input
  rho : Constant  Value=1.205
  vMin : MinMax  Function=max  Inputs=2  SaturateOnIntegerOverflow=on  InputSameDT=on
  F_D : Outport
  PT.nEngine : Outport  Port=2
  wires:
  Sign/1 -> braking force/3
  Product2/1 -> PT.nEngine/1
  vMin/1 -> Product2/1
  Constant1/1 -> vMin/2
  Car.vx_1/1 -> Sign/1, Product4/1, Product4/2, vMin/1
  DM.Brake/1 -> mu/1
  "F_Mmax "/1 -> Product/2
  Look-Up Table/1 -> Product1/3
  Product1/1 -> Product/1, Product2/2
  Constant4/1 -> Product1/1
  Constant3/1 -> Product1/2
  Product/1 -> Sum/1
  DM.GearNo/1 -> Look-Up Table/1
  Sum/1 -> F_D/1
  braking force/1 -> Sum/2
  g/1 -> braking force/2
  m/1 -> g/1
  mu/1 -> braking force/1
  DM.Gas/1 -> "F_Mmax "/1
  A/1 -> Product3/5
  rho/1 -> Product3/4
  Constant6/1 -> Product3/3
  cW/1 -> Product3/2
  Product4/1 -> Product3/1
  Product3/1 -> Sum/3

== system SingleTrack/CarMaker/Vehicle/User Vehicle (CM4SL)/CarAndTrailer/single-track mass point model/yaw ==
  Steer.Ang : Inport
  Car.v : Inport  Port=2
  Car.v_dot : Inport  Port=3
  Car.mass : Inport  Port=4
  1/ J : Gain  Gain=1/1322.5  SaturateOnIntegerOverflow=on  OutDataTypeStr=Inherit: Same as input  ParamDataTypeStr=Inherit: Same as input
  Bus Selector : BusSelector  OutputSignals=Vhcl Cfg Yaw
  Multiply : Product  Inputs=**  OutDataTypeStr=double
  Sum : Sum  Inputs=+-  SaturateOnIntegerOverflow=on  InputSameDT=on  OutDataTypeStr=Inherit: Same as first input
  Sum1 : Sum  SaturateOnIntegerOverflow=on  InputSameDT=on  OutDataTypeStr=Inherit: Same as first input
  Vehicle Initial Cfg : Subsystem  mask(Vehicle Initial Configuration Values){}
      mask help: Provides some initial vehicle configuration values.
  aYaw * dt : Integrator  ExternalReset=level
  side forces : Subsystem
  sideslip angle : Subsystem
  vYaw * dt : Integrator  ExternalReset=level  InitialConditionSource=external
  beta : Outport
  beta_dot : Outport  Port=2
  Car.Yaw : Outport  Port=3
  Car.Yawp : Outport  Port=4
  Car.Yawpp : Outport  Port=5
  Car.Whl.F.SideSlip : Outport  Port=6
  Car.Whl.SideSlip : Outport  Port=7
  wires:
  Bus Selector/1 -> vYaw * dt/3  "<Vhcl Cfg Yaw>"
  side forces/6(alpha_R) -> Car.Whl.SideSlip/1
  side forces/5(alpha_F) -> Car.Whl.F.SideSlip/1
  sideslip angle/1(beta_dot) -> beta_dot/1
  Steer.Ang/1 -> side forces/4(StWhlAngle)
  sideslip angle/2(beta) -> beta/1, side forces/2(beta)
  Car.mass/1 -> sideslip angle/2(m)
  Car.v_dot/1 -> sideslip angle/3(v_dot)
  Sum1/1 -> sideslip angle/5(S)
  Sum/1 -> 1/ J/1
  side forces/1(S_F * l_F) -> Sum/1
  side forces/2(S_R * l_R) -> Sum/2
  1/ J/1 -> Car.Yawpp/1, aYaw * dt/1
  side forces/3(S_V) -> Sum1/1
  side forces/4(S_R) -> Sum1/2
  Car.v/1 -> sideslip angle/4(v), side forces/3(v)
  vYaw * dt/1 -> Car.Yaw/1
  Multiply/1 -> side forces/1(vYaw), sideslip angle/1(vYaw), vYaw * dt/1, Car.Yawp/1
  [TRStart] -> vYaw * dt/2, aYaw * dt/2
  aYaw * dt/1 -> Multiply/2
  [TRSim] -> Multiply/1
  Vehicle Initial Cfg/1(Vhcl.Cfg) -> Bus Selector/1

== system SingleTrack/CarMaker/Vehicle/User Vehicle (ModelMgr)/CarAndTrailer/CarAndTrailerUpd/CreateBus Brake.IF.In ==
  In : Inport
  BusCreator : BusCreator  Inputs=9
  Demux : Demux  Outputs=9
  Out : Outport
  wires:
  Demux/9 -> BusCreator/9  "Brake IF Trq_Reg RR"
  Demux/8 -> BusCreator/8  "Brake IF Trq_Reg RL"
  Demux/7 -> BusCreator/7  "Brake IF Trq_Reg FR"
  Demux/6 -> BusCreator/6  "Brake IF Trq_Reg FL"
  Demux/5 -> BusCreator/5  "Brake IF Trq_Reg_max RR"
  Demux/4 -> BusCreator/4  "Brake IF Trq_Reg_max RL"
  Demux/3 -> BusCreator/3  "Brake IF Trq_Reg_max FR"
  Demux/2 -> BusCreator/2  "Brake IF Trq_Reg_max FL"
  Demux/1 -> BusCreator/1  "Brake IF T_env"
  BusCreator/1 -> Out/1
  In/1 -> Demux/1

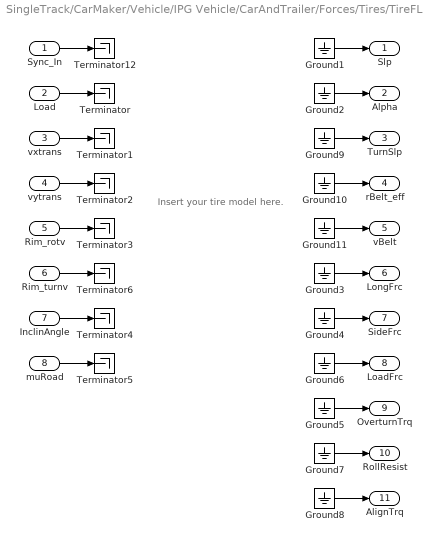
== system SingleTrack/CarMaker/Vehicle/IPG Vehicle/CarAndTrailer/Forces/Tires/TireFL ==
  note: Insert your tire model here.
  Sync_In : Inport
  Load : Inport  Port=2
  vxtrans : Inport  Port=3
  vytrans : Inport  Port=4
  Rim_rotv : Inport  Port=5
  Rim_turnv : Inport  Port=6
  InclinAngle : Inport  Port=7
  muRoad : Inport  Port=8
  Ground{1..11} (11 alike) : Ground
  Terminator{,1..6,12} (8 alike) : Terminator
  Slp : Outport
  Alpha : Outport  Port=2
  TurnSlp : Outport  Port=3
  rBelt_eff : Outport  Port=4
  vBelt : Outport  Port=5
  LongFrc : Outport  Port=6
  SideFrc : Outport  Port=7
  LoadFrc : Outport  Port=8
  OverturnTrq : Outport  Port=9
  RollResist : Outport  Port=10
  AlignTrq : Outport  Port=11
  wires:
  Ground11/1 -> vBelt/1
  Ground10/1 -> rBelt_eff/1
  Ground9/1 -> TurnSlp/1
  Rim_turnv/1 -> Terminator6/1
  Sync_In/1 -> Terminator12/1
  Ground2/1 -> Alpha/1
  Ground3/1 -> LongFrc/1
  Ground4/1 -> SideFrc/1
  Ground5/1 -> OverturnTrq/1
  vxtrans/1 -> Terminator1/1
  vytrans/1 -> Terminator2/1
  Rim_rotv/1 -> Terminator3/1
  InclinAngle/1 -> Terminator4/1
  muRoad/1 -> Terminator5/1
  Load/1 -> Terminator/1
  Ground1/1 -> Slp/1
  Ground6/1 -> LoadFrc/1
  Ground7/1 -> RollResist/1
  Ground8/1 -> AlignTrq/1

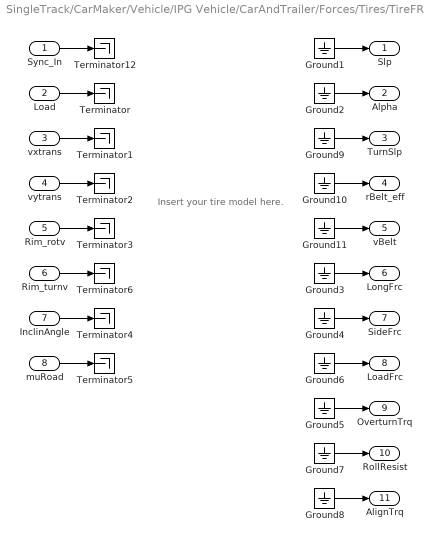
== system SingleTrack/CarMaker/Vehicle/IPG Vehicle/CarAndTrailer/Forces/Tires/TireFR ==
  note: Insert your tire model here.
  Sync_In : Inport
  Load : Inport  Port=2
  vxtrans : Inport  Port=3
  vytrans : Inport  Port=4
  Rim_rotv : Inport  Port=5
  Rim_turnv : Inport  Port=6
  InclinAngle : Inport  Port=7
  muRoad : Inport  Port=8
  Ground{1..11} (11 alike) : Ground
  Terminator{,1..6,12} (8 alike) : Terminator
  Slp : Outport
  Alpha : Outport  Port=2
  TurnSlp : Outport  Port=3
  rBelt_eff : Outport  Port=4
  vBelt : Outport  Port=5
  LongFrc : Outport  Port=6
  SideFrc : Outport  Port=7
  LoadFrc : Outport  Port=8
  OverturnTrq : Outport  Port=9
  RollResist : Outport  Port=10
  AlignTrq : Outport  Port=11
  wires:
  Ground11/1 -> vBelt/1
  Ground10/1 -> rBelt_eff/1
  Ground9/1 -> TurnSlp/1
  Rim_turnv/1 -> Terminator6/1
  Sync_In/1 -> Terminator12/1
  Ground2/1 -> Alpha/1
  Ground3/1 -> LongFrc/1
  Ground4/1 -> SideFrc/1
  Ground5/1 -> OverturnTrq/1
  vxtrans/1 -> Terminator1/1
  vytrans/1 -> Terminator2/1
  Rim_rotv/1 -> Terminator3/1
  InclinAngle/1 -> Terminator4/1
  muRoad/1 -> Terminator5/1
  Load/1 -> Terminator/1
  Ground1/1 -> Slp/1
  Ground6/1 -> LoadFrc/1
  Ground7/1 -> RollResist/1
  Ground8/1 -> AlignTrq/1

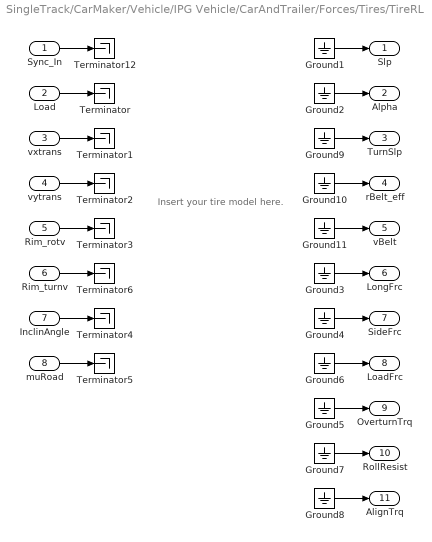
== system SingleTrack/CarMaker/Vehicle/IPG Vehicle/CarAndTrailer/Forces/Tires/TireRL ==
  note: Insert your tire model here.
  Sync_In : Inport
  Load : Inport  Port=2
  vxtrans : Inport  Port=3
  vytrans : Inport  Port=4
  Rim_rotv : Inport  Port=5
  Rim_turnv : Inport  Port=6
  InclinAngle : Inport  Port=7
  muRoad : Inport  Port=8
  Ground{1..11} (11 alike) : Ground
  Terminator{,1..6,12} (8 alike) : Terminator
  Slp : Outport
  Alpha : Outport  Port=2
  TurnSlp : Outport  Port=3
  rBelt_eff : Outport  Port=4
  vBelt : Outport  Port=5
  LongFrc : Outport  Port=6
  SideFrc : Outport  Port=7
  LoadFrc : Outport  Port=8
  OverturnTrq : Outport  Port=9
  RollResist : Outport  Port=10
  AlignTrq : Outport  Port=11
  wires:
  Ground11/1 -> vBelt/1
  Ground10/1 -> rBelt_eff/1
  Ground9/1 -> TurnSlp/1
  Rim_turnv/1 -> Terminator6/1
  Sync_In/1 -> Terminator12/1
  Ground2/1 -> Alpha/1
  Ground3/1 -> LongFrc/1
  Ground4/1 -> SideFrc/1
  Ground5/1 -> OverturnTrq/1
  vxtrans/1 -> Terminator1/1
  vytrans/1 -> Terminator2/1
  Rim_rotv/1 -> Terminator3/1
  InclinAngle/1 -> Terminator4/1
  muRoad/1 -> Terminator5/1
  Load/1 -> Terminator/1
  Ground1/1 -> Slp/1
  Ground6/1 -> LoadFrc/1
  Ground7/1 -> RollResist/1
  Ground8/1 -> AlignTrq/1

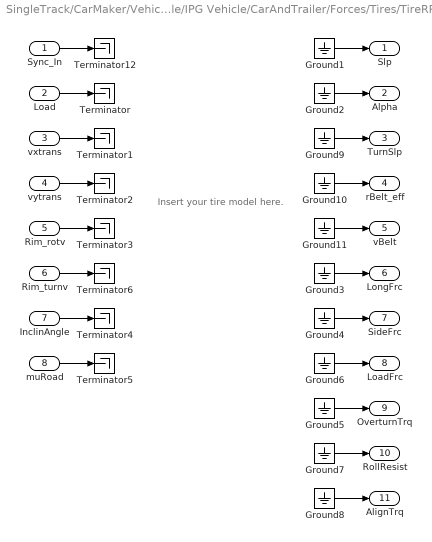
== system SingleTrack/CarMaker/Vehicle/IPG Vehicle/CarAndTrailer/Forces/Tires/TireRR ==
  note: Insert your tire model here.
  Sync_In : Inport
  Load : Inport  Port=2
  vxtrans : Inport  Port=3
  vytrans : Inport  Port=4
  Rim_rotv : Inport  Port=5
  Rim_turnv : Inport  Port=6
  InclinAngle : Inport  Port=7
  muRoad : Inport  Port=8
  Ground{1..11} (11 alike) : Ground
  Terminator{,1..6,12} (8 alike) : Terminator
  Slp : Outport
  Alpha : Outport  Port=2
  TurnSlp : Outport  Port=3
  rBelt_eff : Outport  Port=4
  vBelt : Outport  Port=5
  LongFrc : Outport  Port=6
  SideFrc : Outport  Port=7
  LoadFrc : Outport  Port=8
  OverturnTrq : Outport  Port=9
  RollResist : Outport  Port=10
  AlignTrq : Outport  Port=11
  wires:
  Ground11/1 -> vBelt/1
  Ground10/1 -> rBelt_eff/1
  Ground9/1 -> TurnSlp/1
  Rim_turnv/1 -> Terminator6/1
  Sync_In/1 -> Terminator12/1
  Ground2/1 -> Alpha/1
  Ground3/1 -> LongFrc/1
  Ground4/1 -> SideFrc/1
  Ground5/1 -> OverturnTrq/1
  vxtrans/1 -> Terminator1/1
  vytrans/1 -> Terminator2/1
  Rim_rotv/1 -> Terminator3/1
  InclinAngle/1 -> Terminator4/1
  muRoad/1 -> Terminator5/1
  Load/1 -> Terminator/1
  Ground1/1 -> Slp/1
  Ground6/1 -> LoadFrc/1
  Ground7/1 -> RollResist/1
  Ground8/1 -> AlignTrq/1

== system SingleTrack/CarMaker/Vehicle/User Vehicle (CM4SL)/CarAndTrailer/CreateBus Vhcl.Fr1/Tr2Fr0/Subsystem_00 ==
  sincos : Inport
  Bus Selector : BusSelector  OutputSignals=cry,crz
  Product : Product  RndMeth=Zero
  Tr2Fr1_00 : Outport
  wires:
  sincos/1 -> Bus Selector/1
  Product/1 -> Tr2Fr1_00/1
  Bus Selector/1 -> Product/1  "<cry>"
  Bus Selector/2 -> Product/2  "<crz>"

== system SingleTrack/CarMaker/Vehicle/User Vehicle (CM4SL)/CarAndTrailer/CreateBus Vhcl.Fr1/Tr2Fr0/Subsystem_01 ==
  sincos : Inport
  Add : Sum  Inputs=+-
  Bus Selector : BusSelector  OutputSignals=srx,sry,crz,crx,srz
  Product : Product  Inputs=3  RndMeth=Zero
  Product1 : Product  RndMeth=Zero
  Tr2Fr1_01 : Outport
  wires:
  sincos/1 -> Bus Selector/1
  Product/1 -> Add/1
  Product1/1 -> Add/2
  Add/1 -> Tr2Fr1_01/1
  Bus Selector/1 -> Product/1  "<srx>"
  Bus Selector/2 -> Product/2  "<sry>"
  Bus Selector/3 -> Product/3  "<crz>"
  Bus Selector/4 -> Product1/1  "<crx>"
  Bus Selector/5 -> Product1/2  "<srz>"

== system SingleTrack/CarMaker/Vehicle/User Vehicle (CM4SL)/CarAndTrailer/CreateBus Vhcl.Fr1/Tr2Fr0/Subsystem_02 ==
  sincos : Inport
  Add : Sum
  Bus Selector : BusSelector  OutputSignals=crx,sry,crz,srx,srz
  Product : Product  Inputs=3  RndMeth=Zero
  Product1 : Product  RndMeth=Zero
  Tr2Fr1_02 : Outport
  wires:
  Add/1 -> Tr2Fr1_02/1
  Product1/1 -> Add/2
  Product/1 -> Add/1
  sincos/1 -> Bus Selector/1
  Bus Selector/1 -> Product/1  "<crx>"
  Bus Selector/2 -> Product/2  "<sry>"
  Bus Selector/3 -> Product/3  "<crz>"
  Bus Selector/5 -> Product1/2  "<srz>"
  Bus Selector/4 -> Product1/1  "<srx>"

== system SingleTrack/CarMaker/Vehicle/User Vehicle (CM4SL)/CarAndTrailer/CreateBus Vhcl.Fr1/Tr2Fr0/Subsystem_10 ==
  sincos : Inport
  Bus Selector : BusSelector  OutputSignals=cry,srz
  Product : Product  RndMeth=Zero
  Tr2Fr1_10 : Outport
  wires:
  Bus Selector/2 -> Product/2  "<srz>"
  Bus Selector/1 -> Product/1  "<cry>"
  Product/1 -> Tr2Fr1_10/1
  sincos/1 -> Bus Selector/1

== system SingleTrack/CarMaker/Vehicle/User Vehicle (CM4SL)/CarAndTrailer/CreateBus Vhcl.Fr1/Tr2Fr0/Subsystem_11 ==
  sincos : Inport
  Add : Sum
  Bus Selector : BusSelector  OutputSignals=srx,sry,srz,crx,crz
  Product : Product  Inputs=3  RndMeth=Zero
  Product1 : Product  RndMeth=Zero
  Tr2Fr1_11 : Outport
  wires:
  sincos/1 -> Bus Selector/1
  Product/1 -> Add/1
  Product1/1 -> Add/2
  Add/1 -> Tr2Fr1_11/1
  Bus Selector/1 -> Product/1  "<srx>"
  Bus Selector/2 -> Product/2  "<sry>"
  Bus Selector/3 -> Product/3  "<srz>"
  Bus Selector/5 -> Product1/2  "<crz>"
  Bus Selector/4 -> Product1/1  "<crx>"

== system SingleTrack/CarMaker/Vehicle/User Vehicle (CM4SL)/CarAndTrailer/CreateBus Vhcl.Fr1/Tr2Fr0/Subsystem_12 ==
  sincos : Inport
  Add : Sum  Inputs=+-
  Bus Selector : BusSelector  OutputSignals=crx,sry,srz,srx,crz
  Product : Product  Inputs=3  RndMeth=Zero
  Product1 : Product  RndMeth=Zero
  Tr2Fr1_12 : Outport
  wires:
  Add/1 -> Tr2Fr1_12/1
  Product1/1 -> Add/2
  Product/1 -> Add/1
  sincos/1 -> Bus Selector/1
  Bus Selector/1 -> Product/1  "<crx>"
  Bus Selector/2 -> Product/2  "<sry>"
  Bus Selector/3 -> Product/3  "<srz>"
  Bus Selector/5 -> Product1/2  "<crz>"
  Bus Selector/4 -> Product1/1  "<srx>"

== system SingleTrack/CarMaker/Vehicle/User Vehicle (CM4SL)/CarAndTrailer/CreateBus Vhcl.Fr1/Tr2Fr0/Subsystem_20 ==
  sincos : Inport
  Bus Selector : BusSelector  OutputSignals=sry
  Gain : Gain  Gain=-1
  Tr2Fr1_20 : Outport
  wires:
  sincos/1 -> Bus Selector/1
  Gain/1 -> Tr2Fr1_20/1
  Bus Selector/1 -> Gain/1  "<sry>"

== system SingleTrack/CarMaker/Vehicle/User Vehicle (CM4SL)/CarAndTrailer/CreateBus Vhcl.Fr1/Tr2Fr0/Subsystem_21 ==
  sincos : Inport
  Bus Selector : BusSelector  OutputSignals=srx,cry
  Product : Product  RndMeth=Zero
  Tr2Fr1_21 : Outport
  wires:
  sincos/1 -> Bus Selector/1
  Product/1 -> Tr2Fr1_21/1
  Bus Selector/1 -> Product/1  "<srx>"
  Bus Selector/2 -> Product/2  "<cry>"

== system SingleTrack/CarMaker/Vehicle/User Vehicle (CM4SL)/CarAndTrailer/CreateBus Vhcl.Fr1/Tr2Fr0/Subsystem_22 ==
  sincos : Inport
  Bus Selector : BusSelector  OutputSignals=crx,cry
  Product : Product  RndMeth=Zero
  Tr2Fr1_22 : Outport
  wires:
  Product/1 -> Tr2Fr1_22/1
  sincos/1 -> Bus Selector/1
  Bus Selector/1 -> Product/1  "<crx>"
  Bus Selector/2 -> Product/2  "<cry>"

== system SingleTrack/CarMaker/Vehicle/User Vehicle (CM4SL)/CarAndTrailer/CreateBus Vhcl.Fr1/Tr2Fr0/sincos ==
  Car : Inport
  Bus Creator : BusCreator  Inputs=6
  Bus Selector : BusSelector  OutputSignals=Road_Fr1_rx,Road_Fr1_ry,Car_Yaw
  Trigonometric Function : Trigonometry
  Trigonometric Function1 : Trigonometry  Operator=cos
  Trigonometric Function2 : Trigonometry
  Trigonometric Function3 : Trigonometry
  Trigonometric Function4 : Trigonometry  Operator=cos
  Trigonometric Function5 : Trigonometry  Operator=cos
  sincos : Outport
  wires:
  Bus Selector/1 -> Trigonometric Function/1, Trigonometric Function1/1  "<Road_Fr1_rx>"
  Bus Selector/2 -> Trigonometric Function3/1, Trigonometric Function4/1  "<Road_Fr1_ry>"
  Bus Selector/3 -> Trigonometric Function2/1, Trigonometric Function5/1  "<Car_Yaw>"
  Car/1 -> Bus Selector/1
  Trigonometric Function5/1 -> Bus Creator/6  "crz"
  Trigonometric Function4/1 -> Bus Creator/5  "cry"
  Trigonometric Function1/1 -> Bus Creator/4  "crx"
  Trigonometric Function2/1 -> Bus Creator/3  "srz"
  Trigonometric Function3/1 -> Bus Creator/2  "sry"
  Trigonometric Function/1 -> Bus Creator/1  "srx"
  Bus Creator/1 -> sincos/1

== system SingleTrack/CarMaker/Vehicle/User Vehicle (CM4SL)/CarAndTrailer/PowerTrainUpd/Set OperationState/If Action Subsystem ==
  note: If steering wheel angle is zero, OperationState equals to the desired State by VhclOperator,
  note: else the last value is kept.
  In1 : Inport
  Action Port : ActionPort  ActionType=then
  Abs : Abs
  If : If  IfExpression=u1 <= 0.0175
  If Action Subsystem : Subsystem  TreatAsAtomicUnit=on
  If Action Subsystem1 : Subsystem  TreatAsAtomicUnit=on
  Merge : Merge
  Read CM Dict1 : CarMaker4SL/Read CM Dict  xname=VC.Steer.Ang  xsync=off
  Read CM Dict2 : CarMaker4SL/Read CM Dict  xname=Vhcl.OperationState  xsync=off
  Out1 : Outport
  wires:
  Read CM Dict1/1 -> Abs/1
  Abs/1 -> If/1
  If/1 -> If Action Subsystem/Action
  Merge/1 -> Out1/1
  If Action Subsystem/1(Out1) -> Merge/1
  In1/1 -> If Action Subsystem/1(In1)
  If Action Subsystem1/1(Out1) -> Merge/2
  If/2 -> If Action Subsystem1/Action
  Read CM Dict2/1 -> If Action Subsystem1/1(In1)

== system SingleTrack/CarMaker/Vehicle/User Vehicle (CM4SL)/CarAndTrailer/PowerTrainUpd/Set OperationState/If Action Subsystem1 ==
  In1 : Inport
  Action Port : ActionPort  ActionType=else
  Out1 : Outport
  wires:
  In1/1 -> Out1/1

== system SingleTrack/CarMaker/Vehicle/User Vehicle (CM4SL)/CarAndTrailer/single-track mass point model/Car.v_1/PassIfSim ==
  note: Output original value only when simulating,
      | and zero during pre- or postprocessing.
  In1 : Inport
  "   " : Product  SaturateOnIntegerOverflow=on  InputSameDT=on  OutDataTypeStr=Inherit: Same as first input
  Data Type Conversion : DataTypeConversion
  Out1 : Outport
  wires:
  [TRSim] -> Data Type Conversion/1
  "   "/1 -> Out1/1
  Data Type Conversion/1 -> "   "/2
  In1/1 -> "   "/1

== system SingleTrack/CarMaker/Vehicle/User Vehicle (CM4SL)/CarAndTrailer/single-track mass point model/Vehicle Initial Cfg/CreateBus Vhcl.Cfg ==
  In1 : Inport
  Bus Creator : BusCreator  Inputs=13
  Demux : Demux  Outputs=13
  Out1 : Outport
  wires:
  Demux/13 -> Bus Creator/13  "Vhcl Cfg Whl_rotv RR"
  Bus Creator/1 -> Out1/1
  In1/1 -> Demux/1
  Demux/12 -> Bus Creator/12  "Vhcl Cfg Whl_rotv RL"
  Demux/11 -> Bus Creator/11  "Vhcl Cfg Whl_rotv FR"
  Demux/10 -> Bus Creator/10  "Vhcl Cfg Whl_rotv FL"
  Demux/9 -> Bus Creator/9  "SimCore Trailer nTrailers"
  Demux/8 -> Bus Creator/8  "Vhcl Cfg GearBox_rotv_out"
  Demux/7 -> Bus Creator/7  "Vhcl Cfg Engine_rotv"
  Demux/6 -> Bus Creator/6  "Vhcl Cfg Pitch"
  Demux/5 -> Bus Creator/5  "Vhcl Cfg Yaw"
  Demux/4 -> Bus Creator/4  "Vhcl Cfg Roll"
  Demux/2 -> Bus Creator/2  "Vhcl Cfg Fr1_Pos y"
  Demux/1 -> Bus Creator/1  "Vhcl Cfg Fr1_Pos x"
  Demux/3 -> Bus Creator/3  "Vhcl Cfg Fr1_Pos z"

== system SingleTrack/CarMaker/Vehicle/User Vehicle (CM4SL)/CarAndTrailer/single-track mass point model/yaw/Vehicle Initial Cfg ==
  CreateBus Vhcl.Cfg : Subsystem
  VehicleControlUpd : S-Function  FunctionName=cm_initial  SFunctionDeploymentMode=off  EnableBusSupport=off
  Vhcl.Cfg : Outport
  wires:
  VehicleControlUpd/1 -> CreateBus Vhcl.Cfg/1(In1)
  CreateBus Vhcl.Cfg/1(Out1) -> Vhcl.Cfg/1

== system SingleTrack/CarMaker/Vehicle/User Vehicle (CM4SL)/CarAndTrailer/single-track mass point model/yaw/side forces ==
  vYaw : Inport
  beta : Inport  Port=2
  v : Inport  Port=3
  StWhlAngle : Inport  Port=4
  " " : Product  SaturateOnIntegerOverflow=on  InputSameDT=on  OutDataTypeStr=Inherit: Same as first input
  "  " : Product  SaturateOnIntegerOverflow=on  InputSameDT=on  OutDataTypeStr=Inherit: Same as first input
  "            " : Product  SaturateOnIntegerOverflow=on  InputSameDT=on  OutDataTypeStr=Inherit: Same as first input
  "S_R * l_R " : Product  SaturateOnIntegerOverflow=on  InputSameDT=on  OutDataTypeStr=Inherit: Same as first input
  "S_V * l_V " : Product  SaturateOnIntegerOverflow=on  InputSameDT=on  OutDataTypeStr=Inherit: Same as first input
  Subsystem : Subsystem
  Sum : Sum  SaturateOnIntegerOverflow=on  InputSameDT=on  OutDataTypeStr=Inherit: Same as first input
  Sum1 : Sum  Inputs=-+  SaturateOnIntegerOverflow=on  InputSameDT=on  OutDataTypeStr=Inherit: Same as first input
  Sum4 : Sum  Inputs=+-  SaturateOnIntegerOverflow=on  InputSameDT=on  OutDataTypeStr=Inherit: Same as first input
  c_alphaR : Gain  Gain=50000  SaturateOnIntegerOverflow=on  OutDataTypeStr=Inherit: Same as input  ParamDataTypeStr=Inherit: Same as input
  front wheel steering lock angle : Subsystem
  l__F : Constant  Value=Car_WhlBaseF
  l__R : Constant  Value=-Car_WhlBaseR
  S_F * l_F : Outport
  S_R * l_R : Outport  Port=2
  S_V : Outport  Port=3
  S_R : Outport  Port=4
  alpha_F : Outport  Port=5
  alpha_R : Outport  Port=6
  wires:
  front wheel steering lock angle/1(c_alphaF) -> "            "/1
  StWhlAngle/1 -> front wheel steering lock angle/1(StWhlAngle)
  "S_R * l_R "/1 -> S_R * l_R/1
  Sum4/1 -> alpha_F/1, "            "/2
  front wheel steering lock angle/2(delta_F) -> Sum4/1
  Sum/1 -> front wheel steering lock angle/2(beta + l_F * vYaw / v), Sum4/2
  v/1 -> Subsystem/1(v)
  vYaw/1 -> Subsystem/2(vYaw)
  "S_V * l_V "/1 -> S_F * l_F/1
  "            "/1 -> S_V/1, "S_V * l_V "/1
  c_alphaR/1 -> S_R/1, "S_R * l_R "/1
  Sum1/1 -> alpha_R/1, c_alphaR/1
  "  "/1 -> Sum/2
  " "/1 -> Sum1/2
  l__R/1 -> "S_R * l_R "/2, " "/2
  Subsystem/1(vYaw/v) -> "  "/2, " "/1
  l__F/1 -> "S_V * l_V "/2, "  "/1
  beta/1 -> Sum/1, Sum1/1

== system SingleTrack/CarMaker/Vehicle/User Vehicle (CM4SL)/CarAndTrailer/single-track mass point model/yaw/sideslip angle ==
  vYaw : Inport
  m : Inport  Port=2
  v_dot : Inport  Port=3
  v : Inport  Port=4
  S : Inport  Port=5
  " " : Product  Inputs=*/  SaturateOnIntegerOverflow=on  InputSameDT=on  OutDataTypeStr=Inherit: Same as first input
  "  " : Product  SaturateOnIntegerOverflow=on  InputSameDT=on  OutDataTypeStr=Inherit: Same as first input
  Subsystem : Subsystem
  Sum2 : Sum  Inputs=+-  SaturateOnIntegerOverflow=on  InputSameDT=on  OutDataTypeStr=Inherit: Same as first input
  beta_dot * dt : Integrator  ExternalReset=level
  beta_dot : Outport
  beta : Outport  Port=2
  wires:
  v/1 -> Subsystem/2(v)
  Subsystem/1(Out1) -> beta_dot/1, beta_dot * dt/1
  vYaw/1 -> Subsystem/1(vYaw)
  Sum2/1 -> Subsystem/3(In3)
  "  "/1 -> Sum2/2
  m/1 -> " "/2
  v_dot/1 -> "  "/1
  " "/1 -> Sum2/1
  S/1 -> " "/1
  beta_dot * dt/1 -> "  "/2, beta/1
  [TRStart] -> beta_dot * dt/2

== system SingleTrack/CarMaker/Vehicle/User Vehicle (CM4SL)/CarAndTrailer/PowerTrainUpd/Set OperationState/If Action Subsystem/If Action Subsystem ==
  In1 : Inport
  Action Port : ActionPort  ActionType=then
  Out1 : Outport
  wires:
  In1/1 -> Out1/1

== system SingleTrack/CarMaker/Vehicle/User Vehicle (CM4SL)/CarAndTrailer/PowerTrainUpd/Set OperationState/If Action Subsystem/If Action Subsystem1 ==
  In1 : Inport
  Action Port : ActionPort  ActionType=else
  Out1 : Outport
  wires:
  In1/1 -> Out1/1
